simulink model "rl_control_nnets_temperature"  (R2019b)
settings: Solver=VariableStepAuto  StartTime=0.0  StopTime=300  RelTol=1e-3  EnableMultiTasking=on
undefined symbols (not defined in the file or in its folder): DiscIntNeverNeededParam
libraries: neural x37, simulink x5, rllib x1
(part 2 of 2)

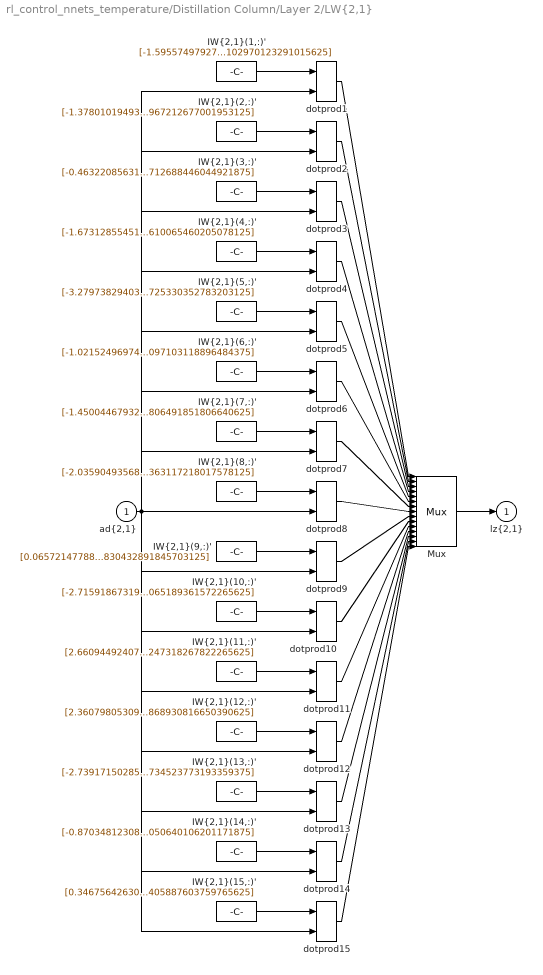
== system rl_control_nnets_temperature/Distillation Column/Layer 2/LW{2,1} ==
  "ad{2,1}" : Inport  PortDimensions=15
      mask Display: e = 0.06;c1 = [120 230 180]/255;c2 = ([120 230 180]+0)/(256+128);c3 = ([120 230 180]+128)/(256+128);patch([0 1 1 0],[0 0 1 1],c1);patch([0 1 1 1-e 1-e 0+e],[0 0 1 1-e 0+e 0+e],c2);patch([0 0 1 1-e 0+e 0+e],[0 1 1 1-e 1-e 0+e],c3);plot([0 1 1 0 0],[0 0 1 1 0]);
  "IW{2,1}(1,:)'" : Constant  Value=[-1.5955749792799343023119718054658733308315277099609375;2.354468933204947322934685871587134897708892822265625;-2.65846408575974368915240120259113609790802001953125;2.06121602608838205838992507779039442539215087890625;-0.97152351453387020274732321922783739864826202392578125;1.4584051750010320613881731333094649016857147216796875;2.7428483784210815343840295099653303623199462890625;0.75528084004964612940824508768855594098567962646484375;0.298859154659074144344543810802861116826534271240234375;-2.051502668815651464484517418895848095417022705078125;1.7886444724494479086018827729276381433010101318359375;-0.2247736926819398350918532969444640912115573883056640625;-2.339913688693712856547790579497814178466796875;-1.0874295567303302600947745304438285529613494873046875;-0.310927544600978988942330261124880053102970123291015625]
      mask Display: e = 0.06;c1 = [120 150 230]/255;c2 = ([120 150 230]+0)/383;c3 = ([120 150 230]+128)/383;patch([0 1 1 0],[0 0 1 1],c1);patch([0 1 1 1-e 1-e 0+e],[0 0 1 1-e 0+e 0+e],c2);patch([0 0 1 1-e 0+e 0+e],[0 1 1 1-e 1-e 0+e],c3);plot([0 1 1 0 0],[0 0 1 1 0]);disp('weights');
  "IW{2,1}(10,:)'" : Constant  Value=[-2.715918673195524934982358900015242397785186767578125;-2.97081158375616194433632699656300246715545654296875;0.048891469782958212053625146609192597679793834686279296875;-0.293966880258761886768326121455174870789051055908203125;-3.029062658385079043199539228226058185100555419921875;-2.480432737091339046031635007238946855068206787109375;1.498148526701775562486318449373356997966766357421875;2.045404346365691683473642115131951868534088134765625;0.333732680638583134591357293174951337277889251708984375;-2.320062078452922893490040223696269094944000244140625;-0.240565119415938333258253578605945222079753875732421875;-0.293769394360880564676108406274579465389251708984375;0.51924927432219403211632879902026616036891937255859375;-1.071800919049726186216275891638360917568206787109375;0.67793390858861446446326226578094065189361572265625]
      mask Display: e = 0.06;c1 = [120 150 230]/255;c2 = ([120 150 230]+0)/383;c3 = ([120 150 230]+128)/383;patch([0 1 1 0],[0 0 1 1],c1);patch([0 1 1 1-e 1-e 0+e],[0 0 1 1-e 0+e 0+e],c2);patch([0 0 1 1-e 0+e 0+e],[0 1 1 1-e 1-e 0+e],c3);plot([0 1 1 0 0],[0 0 1 1 0]);disp('weights');
  "IW{2,1}(11,:)'" : Constant  Value=[2.660944924075097528515243539004586637020111083984375;-1.477918156576268682300678847241215407848358154296875;-1.3964788302237127748384182268637232482433319091796875;0.7025158365675761018565026461146771907806396484375;1.7020084584345240852343295046011917293071746826171875;2.399490896233318348862439961521886289119720458984375;-1.287412747539088631043568966560997068881988525390625;1.43506102469546448219261947087943553924560546875;1.221874124338426792490963634918443858623504638671875;2.871102188598157578525160715798847377300262451171875;-0.87619985000377853534558880710392259061336517333984375;2.089492175712664323583567238529212772846221923828125;0.6497338028738826043451126679428853094577789306640625;-2.1792544378137819194307667203247547149658203125;-0.354740653276739925647831341848359443247318267822265625]
      mask Display: e = 0.06;c1 = [120 150 230]/255;c2 = ([120 150 230]+0)/383;c3 = ([120 150 230]+128)/383;patch([0 1 1 0],[0 0 1 1],c1);patch([0 1 1 1-e 1-e 0+e],[0 0 1 1-e 0+e 0+e],c2);patch([0 0 1 1-e 0+e 0+e],[0 1 1 1-e 1-e 0+e],c3);plot([0 1 1 0 0],[0 0 1 1 0]);disp('weights');
  "IW{2,1}(12,:)'" : Constant  Value=[2.360798053096055948429921045317314565181732177734375;1.3009305335764775879425769744557328522205352783203125;0.9900944782917846520575722024659626185894012451171875;1.265117264773242045095003049937076866626739501953125;-2.31440997815929705438975361175835132598876953125;-1.6976945013427222619384338031522929668426513671875;0.31484632063873652096930300103849731385707855224609375;2.44403108949716152409337155404500663280487060546875;1.66386714295971049892841620021499693393707275390625;-1.5293407765749815752087670261971652507781982421875;1.7927377477131580807423461010330356657505035400390625;-1.0265422771463124096413821462192572653293609619140625;-2.135022501071307754472172746318392455577850341796875;1.971630869477070557849174292641691863536834716796875;1.7909559073544694118851339226239360868930816650390625]
      mask Display: e = 0.06;c1 = [120 150 230]/255;c2 = ([120 150 230]+0)/383;c3 = ([120 150 230]+128)/383;patch([0 1 1 0],[0 0 1 1],c1);patch([0 1 1 1-e 1-e 0+e],[0 0 1 1-e 0+e 0+e],c2);patch([0 0 1 1-e 0+e 0+e],[0 1 1 1-e 1-e 0+e],c3);plot([0 1 1 0 0],[0 0 1 1 0]);disp('weights');
  "IW{2,1}(13,:)'" : Constant  Value=[-2.739171502852727702048696301062591373920440673828125;1.074870554731928162794929448864422738552093505859375;-0.44590916777740030596532960771583020687103271484375;2.295149295723871052388176394742913544178009033203125;0.84688937500738281638490434488630853593349456787109375;2.363273093610308794865204617963172495365142822265625;1.8851135943562040697685233681113459169864654541015625;-0.918180700762579515838979205000214278697967529296875;0.911492537465723895451219505048356950283050537109375;-0.414098915040988002633781661643297411501407623291015625;0.54751591440900126972479711184860207140445709228515625;-2.914059787972651083265418492374010384082794189453125;-2.359798364383767665941604718682356178760528564453125;0.4805722990195404609181650812388397753238677978515625;-2.131651754911300766792692229500971734523773193359375]
      mask Display: e = 0.06;c1 = [120 150 230]/255;c2 = ([120 150 230]+0)/383;c3 = ([120 150 230]+128)/383;patch([0 1 1 0],[0 0 1 1],c1);patch([0 1 1 1-e 1-e 0+e],[0 0 1 1-e 0+e 0+e],c2);patch([0 0 1 1-e 0+e 0+e],[0 1 1 1-e 1-e 0+e],c3);plot([0 1 1 0 0],[0 0 1 1 0]);disp('weights');
  "IW{2,1}(14,:)'" : Constant  Value=[-0.87034812308581310791311125285574235022068023681640625;2.727769776060152029373284676694311201572418212890625;2.204455870313811516325586126185953617095947265625;1.398009701959704642604265245608985424041748046875;2.946927404448183462903898544027470052242279052734375;2.074033329983010265351595080574043095111846923828125;1.502394469776598295851499642594717442989349365234375;0.456353945245641823280635662740678526461124420166015625;0.6210093777171430406980334737454541027545928955078125;-1.4520783874390443823898522168747149407863616943359375;-1.700840584991133663805840114946477115154266357421875;-0.9809760748986686706984983175061643123626708984375;0.732086019481444250089907654910348355770111083984375;1.6870912778977060764162843042868189513683319091796875;2.118716788756398017312676529400050640106201171875]
      mask Display: e = 0.06;c1 = [120 150 230]/255;c2 = ([120 150 230]+0)/383;c3 = ([120 150 230]+128)/383;patch([0 1 1 0],[0 0 1 1],c1);patch([0 1 1 1-e 1-e 0+e],[0 0 1 1-e 0+e 0+e],c2);patch([0 0 1 1-e 0+e 0+e],[0 1 1 1-e 1-e 0+e],c3);plot([0 1 1 0 0],[0 0 1 1 0]);disp('weights');
  "IW{2,1}(15,:)'" : Constant  Value=[0.346756426306968956740917064962559379637241363525390625;0.3972245927880024840561645760317333042621612548828125;-1.07189264310200815799589690868742763996124267578125;-2.160590411509892394548160154954530298709869384765625;2.342780391112710969281351935933344066143035888671875;2.148631237947001171306737887789495289325714111328125;-2.045599711805168308131896992563270032405853271484375;-2.738550877481289891335336506017483770847320556640625;-1.938385462081199772654827029327861964702606201171875;-0.203388778224261213001256010102224536240100860595703125;1.360727229208832600448886296362616121768951416015625;0.53388872810392928869305251282639801502227783203125;-1.5612987099935777823844773593009449541568756103515625;-1.5294814368862790221470504548051394522190093994140625;2.697160710293977192719694357947446405887603759765625]
      mask Display: e = 0.06;c1 = [120 150 230]/255;c2 = ([120 150 230]+0)/383;c3 = ([120 150 230]+128)/383;patch([0 1 1 0],[0 0 1 1],c1);patch([0 1 1 1-e 1-e 0+e],[0 0 1 1-e 0+e 0+e],c2);patch([0 0 1 1-e 0+e 0+e],[0 1 1 1-e 1-e 0+e],c3);plot([0 1 1 0 0],[0 0 1 1 0]);disp('weights');
  "IW{2,1}(2,:)'" : Constant  Value=[-1.378010194938477983583879904472269117832183837890625;-1.3100380751342719509722201109980233013629913330078125;1.9919724587248366365344054429442621767520904541015625;2.51778532771804730572284825029782950878143310546875;-0.90658251338869144664300847580307163298130035400390625;-2.011776230446922664185649409773759543895721435546875;-1.4620381668167932165403044564300216734409332275390625;1.030361403147751264697262740810401737689971923828125;0.623931573627463986753127755946479737758636474609375;-2.325976251075946521496007335372269153594970703125;2.541124287853688823446418609819374978542327880859375;2.209317879951786522951806546188890933990478515625;0.90976454110284044052292529158876277506351470947265625;1.7446798992723115961922530914307571947574615478515625;-1.416596010514443282346519481507129967212677001953125]
      mask Display: e = 0.06;c1 = [120 150 230]/255;c2 = ([120 150 230]+0)/383;c3 = ([120 150 230]+128)/383;patch([0 1 1 0],[0 0 1 1],c1);patch([0 1 1 1-e 1-e 0+e],[0 0 1 1-e 0+e 0+e],c2);patch([0 0 1 1-e 0+e 0+e],[0 1 1 1-e 1-e 0+e],c3);plot([0 1 1 0 0],[0 0 1 1 0]);disp('weights');
  "IW{2,1}(3,:)'" : Constant  Value=[-0.46322085631662412996689681676798500120639801025390625;-1.785346142670814373332177638076245784759521484375;-0.70807791569030575917764736004755832254886627197265625;-0.3622973057963083665100612051901407539844512939453125;-0.009707825477469934905005999326021992601454257965087890625;2.0642735790969961584551128908060491085052490234375;2.195960047597717679224160747253336012363433837890625;-2.106484352087186540103402876411564648151397705078125;0.54983199135906957177866161146084778010845184326171875;-1.5801168069626492229673431211267597973346710205078125;3.1506370536415619909575980273075401782989501953125;0.0063341434213456983270962297183359623886644840240478515625;-0.278376663839984106463276702925213612616062164306640625;2.73863478172656638065518563962541520595550537109375;-2.609252573969917943230711898650042712688446044921875]
      mask Display: e = 0.06;c1 = [120 150 230]/255;c2 = ([120 150 230]+0)/383;c3 = ([120 150 230]+128)/383;patch([0 1 1 0],[0 0 1 1],c1);patch([0 1 1 1-e 1-e 0+e],[0 0 1 1-e 0+e 0+e],c2);patch([0 0 1 1-e 0+e 0+e],[0 1 1 1-e 1-e 0+e],c3);plot([0 1 1 0 0],[0 0 1 1 0]);disp('weights');
  "IW{2,1}(4,:)'" : Constant  Value=[-1.67312855451810182927374626160599291324615478515625;1.7620416086065604499566461527138017117977142333984375;-0.365799717590062412053697471492341719567775726318359375;1.822803587351874643474047843483276665210723876953125;-1.9163476528524097108885371198994107544422149658203125;0.44620327122587222223870639936649240553379058837890625;-0.96289697031777732316726314820698462426662445068359375;2.17666330190417145473702476010657846927642822265625;-1.82379517869948326591611476032994687557220458984375;-0.5166595699810603292689847876317799091339111328125;-2.536793946535356614191414337255991995334625244140625;-2.10604160896355008247837758972309529781341552734375;-1.665892407837098243561513299937359988689422607421875;2.072882157783539458506538721849210560321807861328125;-2.181520423073998404817075424944050610065460205078125]
      mask Display: e = 0.06;c1 = [120 150 230]/255;c2 = ([120 150 230]+0)/383;c3 = ([120 150 230]+128)/383;patch([0 1 1 0],[0 0 1 1],c1);patch([0 1 1 1-e 1-e 0+e],[0 0 1 1-e 0+e 0+e],c2);patch([0 0 1 1-e 0+e 0+e],[0 1 1 1-e 1-e 0+e],c3);plot([0 1 1 0 0],[0 0 1 1 0]);disp('weights');
  "IW{2,1}(5,:)'" : Constant  Value=[-3.2797382940302686193945191917009651660919189453125;0.8293677116322648590340804730658419430255889892578125;0.65129062858135056135466811610967852175235748291015625;-1.6424801859396425118831075451453216373920440673828125;-1.854708675811705287372888051322661340236663818359375;-2.14457388398670811824331394745968282222747802734375;-2.542930041380555561403298270306549966335296630859375;-1.0774238357811309896305829170159995555877685546875;1.7581171150407068903831486750277690589427947998046875;-1.1161271772496605958480131448595784604549407958984375;0.60400103367660717967879691059351898729801177978515625;-2.2264683332947026173087579081766307353973388671875;0.967462685417452394887050104443915188312530517578125;-2.673761127322285435781168416724540293216705322265625;-0.769060738526360143652027545613236725330352783203125]
      mask Display: e = 0.06;c1 = [120 150 230]/255;c2 = ([120 150 230]+0)/383;c3 = ([120 150 230]+128)/383;patch([0 1 1 0],[0 0 1 1],c1);patch([0 1 1 1-e 1-e 0+e],[0 0 1 1-e 0+e 0+e],c2);patch([0 0 1 1-e 0+e 0+e],[0 1 1 1-e 1-e 0+e],c3);plot([0 1 1 0 0],[0 0 1 1 0]);disp('weights');
  "IW{2,1}(6,:)'" : Constant  Value=[-1.0215249697424269026413412575493566691875457763671875;-0.37174646932455501779912765414337627589702606201171875;-0.82105871023172249945076828225865028798580169677734375;1.9317297198439831173999436941812746226787567138671875;1.5166207705685141871043697392451576888561248779296875;-2.28385448207235430828632161137647926807403564453125;1.20725535808224737621685562771745026111602783203125;-2.256691231977626888038912511547096073627471923828125;-2.12694270441171084939924185164272785186767578125;-1.1483369798165714570359341450966894626617431640625;-2.56272391520546083398812697851099073886871337890625;1.741477955169006275326637478428892791271209716796875;-2.037091735324789709693504846654832363128662109375;-2.666728182381799872047167809796519577503204345703125;-0.155429470842411932007820496437489055097103118896484375]
      mask Display: e = 0.06;c1 = [120 150 230]/255;c2 = ([120 150 230]+0)/383;c3 = ([120 150 230]+128)/383;patch([0 1 1 0],[0 0 1 1],c1);patch([0 1 1 1-e 1-e 0+e],[0 0 1 1-e 0+e 0+e],c2);patch([0 0 1 1-e 0+e 0+e],[0 1 1 1-e 1-e 0+e],c3);plot([0 1 1 0 0],[0 0 1 1 0]);disp('weights');
  "IW{2,1}(7,:)'" : Constant  Value=[-1.4500446793287864455379576611449010670185089111328125;-1.07085889865140249099795255460776388645172119140625;2.8062032946617296857994006131775677204132080078125;-2.490900362687743285761143852141685783863067626953125;-1.4062603321133180234170367839396931231021881103515625;1.7824678901311703516086026866105385124683380126953125;-0.96943267265891253092746637776144780218601226806640625;1.0771819222603309373909041823935694992542266845703125;1.2345624331443516563666662477771751582622528076171875;1.208839308932030842669291814672760665416717529296875;0.286986234293394038008528923455742187798023223876953125;0.051603933265938033148056973686834680847823619842529296875;2.7143614108370588411389690008945763111114501953125;-1.7257105343180374479317151781287975609302520751953125;2.847223788330810467783749118098057806491851806640625]
      mask Display: e = 0.06;c1 = [120 150 230]/255;c2 = ([120 150 230]+0)/383;c3 = ([120 150 230]+128)/383;patch([0 1 1 0],[0 0 1 1],c1);patch([0 1 1 1-e 1-e 0+e],[0 0 1 1-e 0+e 0+e],c2);patch([0 0 1 1-e 0+e 0+e],[0 1 1 1-e 1-e 0+e],c3);plot([0 1 1 0 0],[0 0 1 1 0]);disp('weights');
  "IW{2,1}(8,:)'" : Constant  Value=[-2.03590493568961239390091577661223709583282470703125;2.551244787127666224790800697519443929195404052734375;0.5501534323046082253227950786822475492954254150390625;1.856192324994713427344095180160365998744964599609375;-0.8712311446890368404893933984567411243915557861328125;-1.6252125157023991075533331240876577794551849365234375;-2.255667541869293746259472754900343716144561767578125;0.39366308340405276045004256957327015697956085205078125;0.14235485802781122632865162813686765730381011962890625;2.43420486907966893141974651371128857135772705078125;1.9744297749168200351022051108884625136852264404296875;-2.730802158551701719346738173044286668300628662109375;1.5614215368604791311923918328830040991306304931640625;-0.7118538718466147496855001008952967822551727294921875;1.26688324083405223774434489314444363117218017578125]
      mask Display: e = 0.06;c1 = [120 150 230]/255;c2 = ([120 150 230]+0)/383;c3 = ([120 150 230]+128)/383;patch([0 1 1 0],[0 0 1 1],c1);patch([0 1 1 1-e 1-e 0+e],[0 0 1 1-e 0+e 0+e],c2);patch([0 0 1 1-e 0+e 0+e],[0 1 1 1-e 1-e 0+e],c3);plot([0 1 1 0 0],[0 0 1 1 0]);disp('weights');
  "IW{2,1}(9,:)'" : Constant  Value=[0.0657214778873078386833839203973184339702129364013671875;-1.3016412395265881674077945717726834118366241455078125;2.658359555934461493365006390376947820186614990234375;-0.52232556133090801697704819162026979029178619384765625;-1.1175478749534695221967695033526979386806488037109375;-2.1636907020344811058976119966246187686920166015625;1.278269854323642817917061620391905307769775390625;-1.8936149245132016805115426905103959143161773681640625;-0.0003758074972402443425512075236838427372276782989501953125;2.72324545697717468328846734948456287384033203125;-1.08520992455633358275690625305287539958953857421875;2.654846192566049811745187980704940855503082275390625;2.300390196389816566124864039011299610137939453125;0.05707808542156338205142418473769794218242168426513671875;-2.11225136279628333824121000361628830432891845703125]
      mask Display: e = 0.06;c1 = [120 150 230]/255;c2 = ([120 150 230]+0)/383;c3 = ([120 150 230]+128)/383;patch([0 1 1 0],[0 0 1 1],c1);patch([0 1 1 1-e 1-e 0+e],[0 0 1 1-e 0+e 0+e],c2);patch([0 0 1 1-e 0+e 0+e],[0 1 1 1-e 1-e 0+e],c3);plot([0 1 1 0 0],[0 0 1 1 0]);disp('weights');
  Mux : Mux  Inputs=15
      mask Display: e = 0.06;c1 = [120 150 230]/255;c2 = ([120 150 230]+0)/383;c3 = ([120 150 230]+128)/383;patch([0 1 1 0],[0 0 1 1],c1);patch([0 1 1 1-e 1-e 0+e],[0 0 1 1-e 0+e 0+e],c2);patch([0 0 1 1-e 0+e 0+e],[0 1 1 1-e 1-e 0+e],c3);plot([0 1 1 0 0],[0 0 1 1 0]);disp('Mux');
  dotprod{1..15} (15 alike) : neural/Weight Functions/dotprod
      settings: SourceProductName=Deep Learning Toolbox
  "lz{2,1}" : Outport
      mask Display: e = 0.06;c1 = [120 230 180]/255;c2 = ([120 230 180]+0)/(256+128);c3 = ([120 230 180]+128)/(256+128);patch([0 1 1 0],[0 0 1 1],c1);patch([0 1 1 1-e 1-e 0+e],[0 0 1 1-e 0+e 0+e],c2);patch([0 0 1 1-e 0+e 0+e],[0 1 1 1-e 1-e 0+e],c3);plot([0 1 1 0 0],[0 0 1 1 0]);
  wires:
  "IW{2,1}(1,:)'"/1 -> dotprod1/1
  "ad{2,1}"/1 -> dotprod1/2, dotprod2/2, dotprod3/2, dotprod4/2, dotprod5/2, dotprod6/2, dotprod7/2, dotprod8/2, dotprod9/2, dotprod10/2, dotprod11/2, dotprod12/2, dotprod13/2, dotprod14/2, dotprod15/2
  dotprod1/1 -> Mux/1
  "IW{2,1}(2,:)'"/1 -> dotprod2/1
  dotprod2/1 -> Mux/2
  "IW{2,1}(3,:)'"/1 -> dotprod3/1
  dotprod3/1 -> Mux/3
  "IW{2,1}(4,:)'"/1 -> dotprod4/1
  dotprod4/1 -> Mux/4
  "IW{2,1}(5,:)'"/1 -> dotprod5/1
  dotprod5/1 -> Mux/5
  "IW{2,1}(6,:)'"/1 -> dotprod6/1
  dotprod6/1 -> Mux/6
  "IW{2,1}(7,:)'"/1 -> dotprod7/1
  dotprod7/1 -> Mux/7
  "IW{2,1}(8,:)'"/1 -> dotprod8/1
  dotprod8/1 -> Mux/8
  "IW{2,1}(9,:)'"/1 -> dotprod9/1
  dotprod9/1 -> Mux/9
  "IW{2,1}(10,:)'"/1 -> dotprod10/1
  dotprod10/1 -> Mux/10
  "IW{2,1}(11,:)'"/1 -> dotprod11/1
  dotprod11/1 -> Mux/11
  "IW{2,1}(12,:)'"/1 -> dotprod12/1
  dotprod12/1 -> Mux/12
  "IW{2,1}(13,:)'"/1 -> dotprod13/1
  dotprod13/1 -> Mux/13
  "IW{2,1}(14,:)'"/1 -> dotprod14/1
  dotprod14/1 -> Mux/14
  "IW{2,1}(15,:)'"/1 -> dotprod15/1
  dotprod15/1 -> Mux/15
  Mux/1 -> "lz{2,1}"/1

== system rl_control_nnets_temperature/Distillation Column/Layer 3/Delays 1 ==
  "p{3}" : Inport  PortDimensions=15
      mask Display: e = 0.06;c1 = [120 230 180]/255;c2 = ([120 230 180]+0)/(256+128);c3 = ([120 230 180]+128)/(256+128);patch([0 1 1 0],[0 0 1 1],c1);patch([0 1 1 1-e 1-e 0+e],[0 0 1 1-e 0+e 0+e],c2);patch([0 0 1 1-e 0+e 0+e],[0 1 1 1-e 1-e 0+e],c3);plot([0 1 1 0 0],[0 0 1 1 0]);
  mux : Mux  Inputs=1
      mask Display: e = 0.06;c1 = [120 150 230]/255;c2 = ([120 150 230]+0)/383;c3 = ([120 150 230]+128)/383;patch([0 1 1 0],[0 0 1 1],c1);patch([0 1 1 1-e 1-e 0+e],[0 0 1 1-e 0+e 0+e],c2);patch([0 0 1 1-e 0+e 0+e],[0 1 1 1-e 1-e 0+e],c3);plot([0 1 1 0 0],[0 0 1 1 0]);disp('Mux')
  "pd{3,2}" : Outport
      mask Display: e = 0.06;c1 = [120 230 180]/255;c2 = ([120 230 180]+0)/(256+128);c3 = ([120 230 180]+128)/(256+128);patch([0 1 1 0],[0 0 1 1],c1);patch([0 1 1 1-e 1-e 0+e],[0 0 1 1-e 0+e 0+e],c2);patch([0 0 1 1-e 0+e 0+e],[0 1 1 1-e 1-e 0+e],c3);plot([0 1 1 0 0],[0 0 1 1 0]);
  wires:
  "p{3}"/1 -> mux/1
  mux/1 -> "pd{3,2}"/1

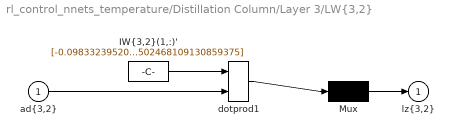
== system rl_control_nnets_temperature/Distillation Column/Layer 3/LW{3,2} ==
  "ad{3,2}" : Inport  PortDimensions=15
      mask Display: e = 0.06;c1 = [120 230 180]/255;c2 = ([120 230 180]+0)/(256+128);c3 = ([120 230 180]+128)/(256+128);patch([0 1 1 0],[0 0 1 1],c1);patch([0 1 1 1-e 1-e 0+e],[0 0 1 1-e 0+e 0+e],c2);patch([0 0 1 1-e 0+e 0+e],[0 1 1 1-e 1-e 0+e],c3);plot([0 1 1 0 0],[0 0 1 1 0]);
  "IW{3,2}(1,:)'" : Constant  Value=[-0.09833239520268226285804047392957727424800395965576171875;-0.466513345489012909439452414517290890216827392578125;0.76658036173321553174986320300376974046230316162109375;-0.352047548007343724663087414228357374668121337890625;-0.87046273113267924603775327341281808912754058837890625;-0.51738999245063943543954110282356850802898406982421875;1.0898086754239304507763108631479553878307342529296875;0.12040186729621842054438474178823526017367839813232421875;0.84265272222510823052488149187411181628704071044921875;-0.93610614681714199303286250142264179885387420654296875;-0.08120884821679395793037059547714306972920894622802734375;-0.3730155367922947107217623852193355560302734375;0.1353604548168242105443681566612212918698787689208984375;-0.461953692748564515024867205283953808248043060302734375;0.9195955317179096422108841579756699502468109130859375]
      mask Display: e = 0.06;c1 = [120 150 230]/255;c2 = ([120 150 230]+0)/383;c3 = ([120 150 230]+128)/383;patch([0 1 1 0],[0 0 1 1],c1);patch([0 1 1 1-e 1-e 0+e],[0 0 1 1-e 0+e 0+e],c2);patch([0 0 1 1-e 0+e 0+e],[0 1 1 1-e 1-e 0+e],c3);plot([0 1 1 0 0],[0 0 1 1 0]);disp('weights');
  Mux : Mux  Inputs=1
      mask Display: e = 0.06;c1 = [120 150 230]/255;c2 = ([120 150 230]+0)/383;c3 = ([120 150 230]+128)/383;patch([0 1 1 0],[0 0 1 1],c1);patch([0 1 1 1-e 1-e 0+e],[0 0 1 1-e 0+e 0+e],c2);patch([0 0 1 1-e 0+e 0+e],[0 1 1 1-e 1-e 0+e],c3);plot([0 1 1 0 0],[0 0 1 1 0]);disp('Mux');
  dotprod1 : neural/Weight Functions/dotprod
      settings: SourceProductName=Deep Learning Toolbox
  "lz{3,2}" : Outport
      mask Display: e = 0.06;c1 = [120 230 180]/255;c2 = ([120 230 180]+0)/(256+128);c3 = ([120 230 180]+128)/(256+128);patch([0 1 1 0],[0 0 1 1],c1);patch([0 1 1 1-e 1-e 0+e],[0 0 1 1-e 0+e 0+e],c2);patch([0 0 1 1-e 0+e 0+e],[0 1 1 1-e 1-e 0+e],c3);plot([0 1 1 0 0],[0 0 1 1 0]);
  wires:
  "IW{3,2}(1,:)'"/1 -> dotprod1/1
  "ad{3,2}"/1 -> dotprod1/2
  dotprod1/1 -> Mux/1
  Mux/1 -> "lz{3,2}"/1
